simulink model "graph_canbang"  (R2022b)
settings: Solver=VariableStepAuto  StartTime=0.0  StopTime=30  RelTol=1e-3
undefined symbols (not defined in the file): A, B, C, C2, D2, Gamma, K1, K2
settings Model: Creator=ASUS  LastModifiedBy=ASUS

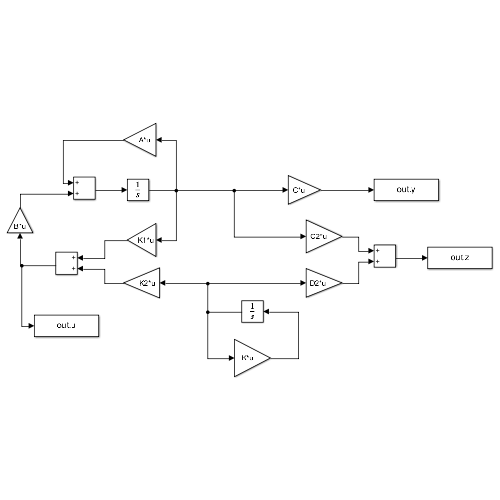
[thumbnail: Simulink's stored preview of the top-level diagram]
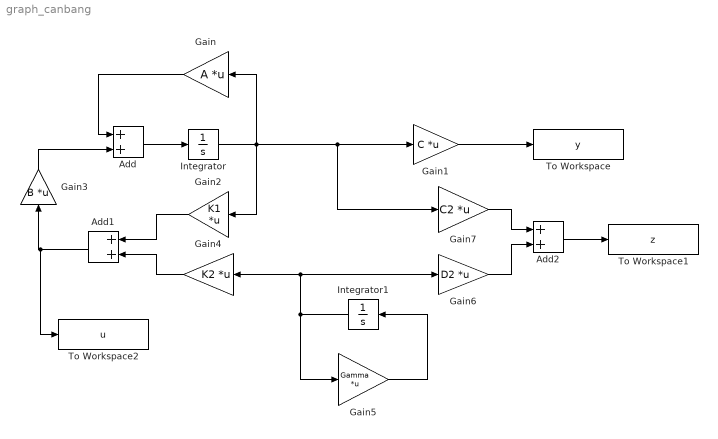
== system graph_canbang ==
  Add : Sum
  Add1 : Sum
  Add2 : Sum
  Gain : Gain  Gain=A  Multiplication=Matrix(K*u)
  Gain1 : Gain  Gain=C  Multiplication=Matrix(K*u)
  Gain2 : Gain  Gain=K1  Multiplication=Matrix(K*u)
  Gain3 : Gain  Gain=B  Multiplication=Matrix(K*u)
  Gain4 : Gain  Gain=K2  Multiplication=Matrix(K*u)
  Gain5 : Gain  Gain=Gamma  Multiplication=Matrix(K*u)
  Gain6 : Gain  Gain=D2  Multiplication=Matrix(K*u)
  Gain7 : Gain  Gain=C2  Multiplication=Matrix(K*u)
  Integrator : Integrator  InitialCondition=[0.1;0.1;0;0]
  Integrator1 : Integrator  InitialCondition=[0;0;0.01;0]
  To Workspace : ToWorkspace  VariableName=y  SaveFormat=Structure With Time  SampleTime=-1
  To Workspace1 : ToWorkspace  VariableName=z  SaveFormat=Structure With Time  SampleTime=-1
  To Workspace2 : ToWorkspace  VariableName=u  SaveFormat=Structure With Time  SampleTime=-1
  wires:
  Add/1 -> Integrator/1
  Gain/1 -> Add/1
  Integrator/1 -> Gain2/1, Gain/1, Gain7/1, Gain1/1
  Gain3/1 -> Add/2
  Gain1/1 -> To Workspace/1
  Gain2/1 -> Add1/1
  Gain4/1 -> Add1/2
  Add1/1 -> To Workspace2/1, Gain3/1
  Gain5/1 -> Integrator1/1
  Integrator1/1 -> Gain5/1, Gain6/1, Gain4/1
  Gain7/1 -> Add2/1
  Gain6/1 -> Add2/2
  Add2/1 -> To Workspace1/1
